simulink model "Controllers_base_FB_2019b"  (R2019b)
settings: Solver=VariableStepAuto  StartTime=0.0  StopTime=10.0  RelTol=1e-3
values from neighbouring files (symbols this model uses):
  sysest_ct = d2c(sysest)    [main.m]
  v_a_max = 10    [main.m]
undefined symbols (not defined in the file or in its folder): HIL, Kp, qc_get_step_size, sigbuilder_block, Ti
libraries: quarc_library x4, cstblocks x3, simulink_extras x3
settings Model: Creator=jesuc  LastModifiedBy=AleFire
settings DataIOCC: SaveFormat=Array  ReturnWorkspaceOutputs=off
settings DebuggingCC: SFMachineParentedDataDiag=error

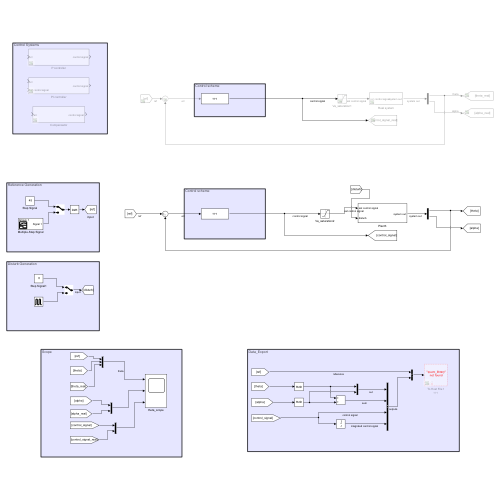
[thumbnail: Simulink's stored preview of the top-level diagram]
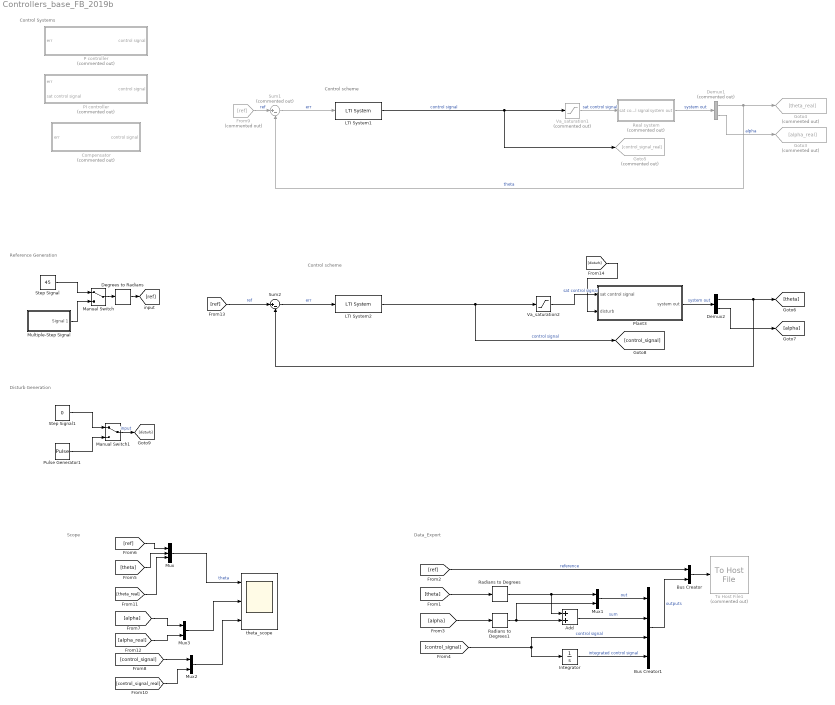
== system Controllers_base_FB_2019b ==
  note: Scope
  note: Control Systems
  note: Reference Generation
  note: Control scheme
  note: Control scheme
  note: Disturb Generation
  note: Data_Export
  Add : Sum
  Bus Creator : BusCreator  Inputs=2
  Bus Creator1 : BusCreator  Inputs=4
  Compensator : Subsystem  Commented=on
  Degrees to Radians : simulink_extras/Transformations/Degrees to Radians
  Demux1 : Demux  Commented=on  Outputs=2
  Demux2 : Demux  Outputs=2
  From9 : From  Commented=on  GotoTag=ref
  Goto3 : Goto  Commented=on  GotoTag=alpha_real
  Goto4 : Goto  Commented=on  GotoTag=theta_real
  Goto5 : Goto  Commented=on  GotoTag=control_signal_real
  Integrator : Integrator
  LTI System1 : cstblocks/LTI System  sys=controller  IC=[]
  LTI System2 : cstblocks/LTI System  sys=controller  IC=[]
  Manual Switch : ManualSwitch
  Manual Switch1 : ManualSwitch
  Multiple-Step Signal : Subsystem  Tag=STV Subsys  LoadFcn=sigbuilder_block('load');  StartFcn=sigbuilder_block('start');  StopFcn=sigbuilder_block('stop');  ClipboardFcn=sigbuilder_block('clipboard');  mask(Sigbuilder block){tuvar=[0:10]}
      mask help: Simulink:masks:SigbuilderBlock_MD
      mask init:
      | if ~strcmp(get_param(bdroot(gcbh),'SimulationStatus'),'stopped') tuvar = sigbuilder_block('maskInit'); end
      settings: CopyFcn=sigbuilder_block('copy');  DeleteFcn=sigbuilder_block('delete');  ModelCloseFcn=sigbuilder_block('modelClose');  PreSaveFcn=sigbuilder_block('preSave');  PauseFcn=sigbuilder_block('pause');  ContinueFcn=sigbuilder_block('continue');  NameChangeFcn=sigbuilder_block('namechange');  OpenFcn=sigbuilder_block('open',[437.6 199.2 550.4 400 ]);  CloseFcn=sigbuilder_block('close');
      mask Display: plot(0, 0, 100, 100,[2, 2, 32, 32, 2], [68, 8, 8, 68, 68],[32, 2], [38, 38], [32, 19, 2],[53, 60, 44], [32, 17, 17, 2],[16, 16, 31, 31]);txt = getActiveGroup(gcbh);text(2, 100, txt,'verticalAlignment', 'top');
  Mux : Mux  Inputs=3
  Mux1 : Mux  Inputs=2
  Mux2 : Mux  Inputs=2
  Mux3 : Mux  Inputs=2
  P controller : Subsystem  Commented=on
  PI controller : Subsystem  Commented=on
  Plant3 : Subsystem
  Pulse Generator1 : DiscretePulseGenerator  PulseType=Time based  Amplitude=.2  Period=1.5  PulseWidth=5
  Radians to Degrees : simulink_extras/Transformations/Radians to Degrees
  Radians to Degrees1 : simulink_extras/Transformations/Radians to Degrees
  Real system : Subsystem  Commented=on
  Step Signal : Constant  Value=45
  Step Signal1 : Constant  Value=0
  Sum1 : Sum  Commented=on  Inputs=|+-
  Sum2 : Sum  Inputs=|+-
  To Host File1 : quarc_library/Sinks/To Host/To Host File  Commented=on  file_name=Sine tests\Sine_24_in_theta_alpha.mat  variable_name=data  decimation=1  sample_time=-1  file_format=MAT-file v.4  options=No header or footer  append=off  final_file_name=Sine tests\Sine_24_in_theta_alpha.mat  bitrate=2000000
  Va_saturation1 : Saturate  Commented=on  UpperLimit=v_a_max  LowerLimit=-v_a_max
  Va_saturation2 : Saturate  UpperLimit=v_a_max  LowerLimit=-v_a_max
  theta_scope : Scope  NumInputPorts=3
  wires:
  Multiple-Step Signal/1(Signal 1) -> Manual Switch/2
  Step Signal/1 -> Manual Switch/1
  Manual Switch/1 -> Degrees to Radians/1
  Mux/1 -> theta_scope/1  "theta"
  Degrees to Radians/1 -> [ref]
  [ref] -> Mux/1
  [theta] -> Mux/2
  [alpha] -> Mux3/1
  Mux2/1 -> theta_scope/3
  Va_saturation1/1 -> Real system/1(sat control signal)  "sat control signal"
  Demux1/1 -> Goto4/1, Sum1/2  "theta"
  Sum1/1 -> LTI System1/1  "err"
  From9/1 -> Sum1/1  "ref"
  Demux1/2 -> Goto3/1  "alpha"
  LTI System1/1 -> Va_saturation1/1, Goto5/1  "control signal"
  Real system/1(system out) -> Demux1/1  "system out"
  [control_signal] -> Mux2/1
  [control_signal_real] -> Mux2/2
  [theta_real] -> Mux/3
  [alpha_real] -> Mux3/2
  Mux3/1 -> theta_scope/2
  Plant3/1(system out) -> Demux2/1  "system out"
  Demux2/1 -> [theta], Sum2/2
  Va_saturation2/1 -> Plant3/1(sat control signal)  "sat control signal"
  Demux2/2 -> [alpha]
  [ref] -> Sum2/1  "ref"
  [disturb] -> Plant3/2(disturb)
  LTI System2/1 -> Va_saturation2/1, [control_signal]  "control signal"
  Sum2/1 -> LTI System2/1  "err"
  Pulse Generator1/1 -> Manual Switch1/2
  Step Signal1/1 -> Manual Switch1/1
  Manual Switch1/1 -> [disturb]  "input"
  [control_signal] -> Integrator/1, Bus Creator1/3  "control signal"
  [alpha] -> Radians to Degrees1/1
  Radians to Degrees1/1 -> Add/2, Mux1/2
  Add/1 -> Bus Creator1/2  "sum"
  Bus Creator1/1 -> Bus Creator/2  "outputs"
  Bus Creator/1 -> To Host File1/1
  [ref] -> Bus Creator/1  "reference"
  Integrator/1 -> Bus Creator1/4  "integrated control signal"
  [theta] -> Radians to Degrees/1
  Radians to Degrees/1 -> Add/1, Mux1/1
  Mux1/1 -> Bus Creator1/1  "out"

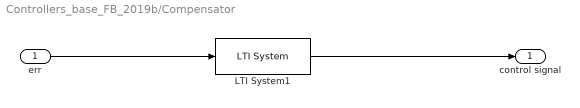
== system Controllers_base_FB_2019b/Compensator ==
  err : Inport
  LTI System1 : cstblocks/LTI System  sys=controller  IC=[]
  control signal : Outport
  wires:
  LTI System1/1 -> control signal/1
  err/1 -> LTI System1/1

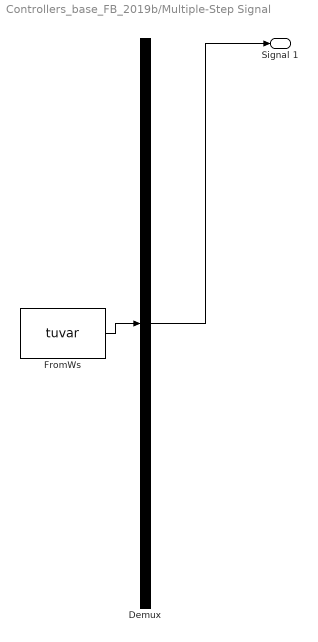
== system Controllers_base_FB_2019b/Multiple-Step Signal ==
  Demux : Demux  Tag=STV Demux  Outputs=1
      settings: DisplayOption=none
  FromWs : FromWorkspace  Tag=STV FromWs  VariableName=tuvar
      SigBuilderData=|
      | common.afterFinalStr = 'Extrapolate'
      | common.sampleTime = 0
      | dataSet.timeRange = [0 10]
      | dataSet.name = 'Group 1'
      | sbobj.Groups.Name = 'Group 1'
      | sbobj.Groups.Signals.Name = 'Signal 1'
      | sbobj.Groups.Signals.XData = [0 1 1 3 3 5 5 7 7 8.5 8.5 10]
      | sbobj.Groups.Signals.YData = [0.005 0.005 40 40 15 15 -30 -30 0 0 23 23]
  Signal 1 : Outport  Tag=STV Outport
  wires:
  Demux/1 -> Signal 1/1
  FromWs/1 -> Demux/1

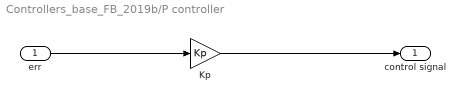
== system Controllers_base_FB_2019b/P controller ==
  err : Inport
  Kp : Gain  Gain=Kp
  control signal : Outport
  wires:
  err/1 -> Kp/1
  Kp/1 -> control signal/1

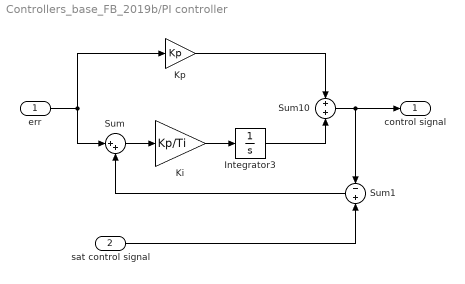
== system Controllers_base_FB_2019b/PI controller ==
  err : Inport
  sat control signal : Inport  Port=2
  Integrator3 : Integrator
  Ki : Gain  Gain=Kp/Ti
  Kp : Gain  Gain=Kp
  Sum : Sum  Inputs=|++
  Sum1 : Sum  Inputs=-+
  Sum10 : Sum
  control signal : Outport
  wires:
  err/1 -> Sum/1, Kp/1
  Ki/1 -> Integrator3/1
  Sum10/1 -> control signal/1, Sum1/1
  Integrator3/1 -> Sum10/2
  Kp/1 -> Sum10/1
  Sum/1 -> Ki/1
  sat control signal/1 -> Sum1/2
  Sum1/1 -> Sum/2

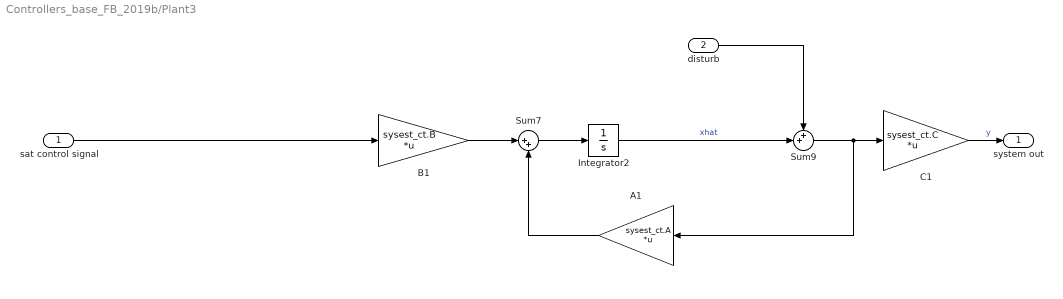
== system Controllers_base_FB_2019b/Plant3 ==
  sat control signal : Inport
  disturb : Inport  Port=2
  A1 : Gain  Gain=sysest_ct.A  Multiplication=Matrix(K*u)
  B1 : Gain  Gain=sysest_ct.B  Multiplication=Matrix(K*u)
  C1 : Gain  Gain=sysest_ct.C  Multiplication=Matrix(K*u)
  Integrator2 : Integrator
  Sum7 : Sum  Inputs=|++
  Sum9 : Sum  Inputs=++|
  system out : Outport
  wires:
  Sum7/1 -> Integrator2/1
  disturb/1 -> Sum9/1
  B1/1 -> Sum7/1
  Integrator2/1 -> Sum9/2  "xhat"
  C1/1 -> system out/1  "y"
  A1/1 -> Sum7/2
  Sum9/1 -> A1/1, C1/1
  sat control signal/1 -> B1/1

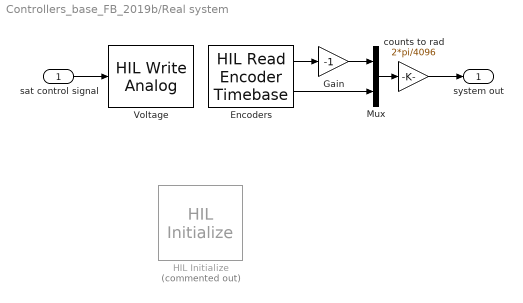
== system Controllers_base_FB_2019b/Real system ==
  sat control signal : Inport
  Encoders : quarc_library/Data Acquisition/Generic/Timebases/HIL Read Encoder Timebase  object_name=HIL-1  clock=0  channels=[0:1]  samples_in_buffer=max(ceil(1/qc_get_step_size), 1)  active=on  vector_output=off  data_type_mode=Inherit via back propagation  data_type=double
  Gain : Gain  Gain=-1
  HIL Initialize : quarc_library/Data Acquisition/Generic/Configuration/HIL Initialize  Priority=-99  Commented=on  object_name=HIL-1  board_type=q2_usb  board_number=0  board_options=d0=digital;d1=digital;led=auto;update_rate=normal;decimation=1  exclusive=off  active=off  hardware_clocks=[0]  clock_modes=[]  initial_clock_frequencies=[]  set_clock_params_at_start=off  set_clock_params_at_switch_in=off  set_clock_frequencies_at_start=off  set_clock_frequencies_at_switch_in=off  analog_input_channels=[0:1]  analog_input_configurations=[]  analog_input_maximums=10  analog_input_minimums=-10  set_analog_input_params_at_start=on  set_analog_input_params_at_switch_in=off  analog_output_channels=[0:1]  analog_output_maximums=10  analog_output_minimums=-10  initial_analog_outputs=[0]  final_analog_outputs=[0]  watchdog_analog_outputs=0  set_analog_output_params_at_start=on  set_analog_output_params_at_switch_in=off  set_analog_outputs_at_start=on  set_analog_outputs_at_switch_in=off  set_analog_outputs_at_terminate=on  set_analog_outputs_at_switch_out=off  set_analog_outputs_on_watchdog=off  digital_input_channels=[]  digital_output_channels=[]  digital_output_configuration=[]  initial_digital_outputs=[1]  final_digital_outputs=[1]  watchdog_digital_outputs=[1]  set_digital_output_params_at_start=off  set_digital_output_params_at_switch_in=off  set_digital_outputs_at_start=on  set_digital_outputs_at_switch_in=off  set_digital_outputs_at_terminate=on  set_digital_outputs_at_switch_out=off  set_digital_outputs_on_watchdog=off  encoder_channels=[0:1]  quadrature=[4]  encoder_filter_frequency=[]  initial_encoder_counts=[0]  set_encoder_params_at_start=on  set_encoder_params_at_switch_in=off  set_encoder_counts_at_start=on  set_encoder_counts_at_switch_in=off  pwm_channels=[]  pwm_modes=[0]  pwm_frequency=1/0.020  pwm_configuration=[]  pwm_alignment=[]  pwm_polarity=[]  pwm_leading_deadband=[]  pwm_trailing_deadband=[]  initial_pwm_outputs=[0]  final_pwm_outputs=[0]  watchdog_pwm_outputs=[0]  set_pwm_params_at_start=on  set_pwm_params_at_switch_in=off  set_pwm_outputs_at_start=on  set_pwm_outputs_at_switch_in=off  set_pwm_outputs_at_terminate=on  set_pwm_outputs_at_switch_out=off  set_pwm_outputs_on_watchdog=off  other_output_channels=[]  initial_other_outputs=[]  final_other_outputs=[]  watchdog_other_outputs=[]  set_other_outputs_at_start=off  set_other_outputs_at_switch_in=off  set_other_outputs_at_terminate=off  set_other_outputs_at_switch_out=off  set_other_outputs_on_watchdog=off
  Mux : Mux  Inputs=2
  Voltage : quarc_library/Data Acquisition/Generic/Immediate I//O/HIL Write Analog  object_name=HIL-1  channels=0  sample_time=-1  active=off  vector_input=off
  counts to rad : Gain  Gain=2*pi/4096
  system out : Outport
  wires:
  sat control signal/1 -> Voltage/1
  Encoders/1 -> Gain/1
  Encoders/2 -> Mux/2
  Mux/1 -> counts to rad/1
  Gain/1 -> Mux/1
  counts to rad/1 -> system out/1
